simulink model "induction_motor_drive"  (Simulink 5.0)
settings: Solver=ode23tb  SolverMode=SingleTasking  StartTime=0.0  StopTime=2  MaxStep=10e-6  RelTol=1e-4
undefined symbols (not defined in the file): sigbuilder_block
libraries: powerlib2 x6
settings Model: Creator=Oros  ExtModeTrigMode=oneshot  ExtModeArmWhenConnect=off  ExternalInput=[]  TimeSaveName=t  SaveOutput=off  LimitDataPoints=off  UnconnectedInputMsg=none  UnconnectedOutputMsg=none  BlockReductionOpt=off  BooleanDataType=off  RTWTemplateMakefile=grt_unix.tmf

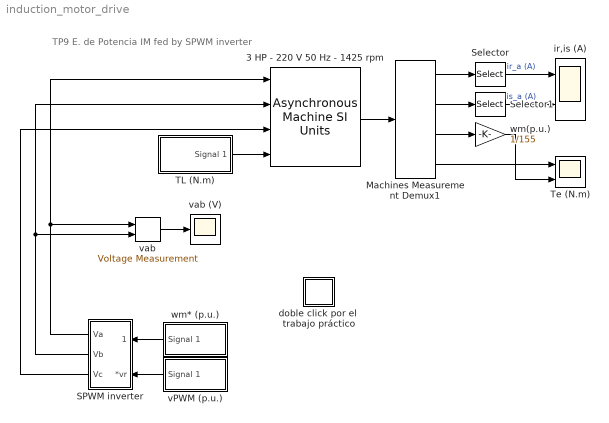
== system induction_motor_drive ==
  note: TP9 E. de Potencia
      | IM fed by SPWM inverter
  3 HP - 220 V 50 Hz - 1425 rpm : powerlib2/Machines/Asynchronous Machine SI Units  Tag=PoWeRsYsTeMbLoCk  rotType=Squirrel-cage  ctrl=Stationary  x1=[ 5*746, 220, 50 ]  x2="[ 0.435  2*2.0e-3 ]"  x3="[ 0.816  2.0e-3 ]"  x4=69.31e-3  x5="[ 0.089  0  2 ]"  x6="[ 1,0   0,0,0   0,0,0 ]"  PSBOutputType=1110  iounits=1  LoadFlowParameters=0
  Machines Measurement Demux1 : powerlib2/Machines/Machines Measurement Demux  machType=Asynchronous  ssm1=on  ssm2=on  ssm3=on  ssm4=on  ssm5=on  ssm6=on  sm1=off  sm2=on  sm3=off  sm4=off  sm5=off  sm6=on  sm7=off  sm8=on  sm9=off  sm10=off  sm11=off  sm115=off  sm12=off  sm13=off  sm14=off  asm1=on  asm2=off  asm3=off  asm4=off  asm5=on  asm6=off  asm7=off  asm8=off  asm9=on  asm10=on  asm11=off  pmsm1=on  pmsm2=on  pmsm3=on  pmsm4=on  pmsm5=on  pmsm6=on  lastType=1
  SPWM inverter : Subsystem  Orientation=left
  Selector : Selector  InputPortWidth=3
  Selector1 : Selector  InputPortWidth=3
  TL (N.m) : Subsystem  Tag=STV Subsys  StartFcn=sigbuilder_block('start');  StopFcn=sigbuilder_block('stop');  ClipboardFcn=sigbuilder_block('clipboard');  mask(Sigbuilder block){}
      mask help: Sigbuilder GUI
      mask init:
      | if ~strcmp(get_param(bdroot(gcb),'SimulationStatus'),'stopped') tuvar = sigbuilder_block('maskInit'); end
      settings: CopyFcn=sigbuilder_block('copy');  DeleteFcn=sigbuilder_block('delete');  ModelCloseFcn=sigbuilder_block('modelClose');  PreSaveFcn=sigbuilder_block('preSave');  NameChangeFcn=sigbuilder_block('namechange');  OpenFcn=sigbuilder_block('open',[78 40.5 391.5 291 ]);  CloseFcn=sigbuilder_block('close');
      mask Display: plot(0,0,100,100,[10,10,40,40,10],[80,20,20,80,80],[40,10],[50,50], [40,27,10],[65,72,56],[40,25,25,10],[28,28,43,43]);
  Te (N.m) : Scope  NumInputPorts=2
      settings: YMin=-125~0.05  YMax=200~1.05  DataFormat=Structure
  doble click por el  trabajo práctico : Subsystem
      mask Display: disp('?')
  ir,is (A) : Scope  NumInputPorts=2
      settings: YMin=-100~-80  YMax=110~100  DataFormat=Structure
  vPWM (p.u.) : Subsystem  Tag=STV Subsys  Orientation=left  StartFcn=sigbuilder_block('start');  StopFcn=sigbuilder_block('stop');  ClipboardFcn=sigbuilder_block('clipboard');  mask(Sigbuilder block){}
      mask help: Sigbuilder GUI
      mask init:
      | if ~strcmp(get_param(bdroot(gcb),'SimulationStatus'),'stopped') tuvar = sigbuilder_block('maskInit'); end
      settings: CopyFcn=sigbuilder_block('copy');  DeleteFcn=sigbuilder_block('delete');  ModelCloseFcn=sigbuilder_block('modelClose');  PreSaveFcn=sigbuilder_block('preSave');  NameChangeFcn=sigbuilder_block('namechange');  OpenFcn=sigbuilder_block('open',[78 40.5 391.5 291 ]);  CloseFcn=sigbuilder_block('close');
      mask Display: plot(0,0,100,100,[10,10,40,40,10],[80,20,20,80,80],[40,10],[50,50], [40,27,10],[65,72,56],[40,25,25,10],[28,28,43,43]);
  vab : powerlib2/Measurements/Voltage Measurement  Tag=PoWeRsYsTeMmEaSuReMeNt  PhasorSimulation=off  OutputType=Magnitude  PSBOutputType=0  PSBequivalent=1
  vab (V) : Scope
      settings: YMin=-400  YMax=400  DataFormat=Structure
  wm(p.u.) : Gain  Gain=1/155  SaturateOnIntegerOverflow=on
  wm* (p.u.) : Subsystem  Tag=STV Subsys  Orientation=left  StartFcn=sigbuilder_block('start');  StopFcn=sigbuilder_block('stop');  ClipboardFcn=sigbuilder_block('clipboard');  mask(Sigbuilder block){}
      mask help: Sigbuilder GUI
      mask init:
      | if ~strcmp(get_param(bdroot(gcb),'SimulationStatus'),'stopped') tuvar = sigbuilder_block('maskInit'); end
      settings: CopyFcn=sigbuilder_block('copy');  DeleteFcn=sigbuilder_block('delete');  ModelCloseFcn=sigbuilder_block('modelClose');  PreSaveFcn=sigbuilder_block('preSave');  NameChangeFcn=sigbuilder_block('namechange');  OpenFcn=sigbuilder_block('open',[78 40.5 391.5 291 ]);  CloseFcn=sigbuilder_block('close');
      mask Display: plot(0,0,100,100,[10,10,40,40,10],[80,20,20,80,80],[40,10],[50,50], [40,27,10],[65,72,56],[40,25,25,10],[28,28,43,43]);
  wires:
  SPWM inverter/1(Va) -> vab/1, 3 HP - 220 V 50 Hz - 1425 rpm/1
  SPWM inverter/2(Vb) -> vab/2, 3 HP - 220 V 50 Hz - 1425 rpm/2
  vab/1 -> vab (V)/1
  Machines Measurement Demux1/1 -> Selector/1
  Machines Measurement Demux1/3 -> wm(p.u.)/1
  Machines Measurement Demux1/4 -> Te (N.m)/1
  Machines Measurement Demux1/2 -> Selector1/1
  Selector/1 -> ir,is (A)/1  "ir_a (A)"
  Selector1/1 -> ir,is (A)/2  "is_a (A)"
  3 HP - 220 V 50 Hz - 1425 rpm/1 -> Machines Measurement Demux1/1
  SPWM inverter/3(Vc) -> 3 HP - 220 V 50 Hz - 1425 rpm/3
  wm* (p.u.)/1(Signal 1) -> SPWM inverter/1(*wr)
  vPWM (p.u.)/1(Signal 1) -> SPWM inverter/2(*vr)
  wm(p.u.)/1 -> Te (N.m)/2
  TL (N.m)/1(Signal 1) -> 3 HP - 220 V 50 Hz - 1425 rpm/4

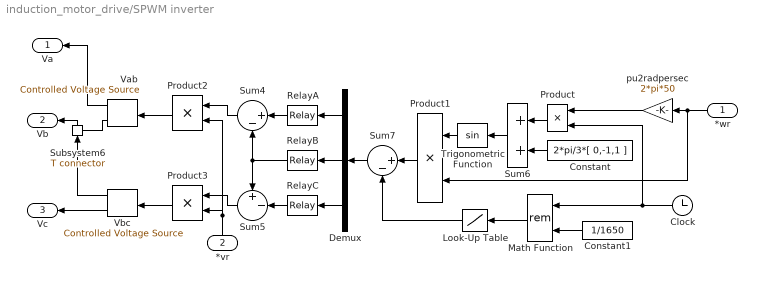
== system induction_motor_drive/SPWM inverter ==
  *wr : Inport  Orientation=left
  *vr : Inport  Orientation=up  Port=2
  Clock : Clock
      settings: Decimation=10
  Constant : Constant  Orientation=left  Value=2*pi/3*[ 0,-1,1 ]
  Constant1 : Constant  Orientation=left  Value=1/1650
  Demux : Demux  Orientation=left  Outputs=3
  Look-Up Table : Lookup  Orientation=left  InputValues="[0 0.25  0.75  1] / 1650"  OutputValues="[0  1  -1  0]"  SaturateOnIntegerOverflow=on
  Math Function : Math  Orientation=left  Operator=rem
  Product : Product  Orientation=left  SaturateOnIntegerOverflow=on  InputSameDT=on
  Product1 : Product  Orientation=left  SaturateOnIntegerOverflow=on  InputSameDT=on
  Product2 : Product  Orientation=left  SaturateOnIntegerOverflow=on
  Product3 : Product  Orientation=left  SaturateOnIntegerOverflow=on
  RelayA : Relay  Orientation=left  OnSwitchValue=0  OffSwitchValue=0  OnOutputValue=220*sqrt(2/3)  OffOutputValue=-220*sqrt(2/3)
  RelayB : Relay  Orientation=left  OnSwitchValue=0  OffSwitchValue=0  OnOutputValue=220*sqrt(2/3)  OffOutputValue=-220*sqrt(2/3)
  RelayC : Relay  Orientation=left  OnSwitchValue=0  OffSwitchValue=0  OnOutputValue=220*sqrt(2/3)  OffOutputValue=-220*sqrt(2/3)
  Subsystem6 : powerlib2/Connectors/T connector  Tag=PoWeRsYsTeMbLoCk  Orientation=up  PSBOutputType=1
  Sum4 : Sum  Orientation=left  Inputs=|+-  SaturateOnIntegerOverflow=on  InputSameDT=on
  Sum5 : Sum  Orientation=left  Inputs=+-|  SaturateOnIntegerOverflow=on  InputSameDT=on
  Sum6 : Sum  Orientation=left  SaturateOnIntegerOverflow=on  InputSameDT=on
  Sum7 : Sum  Orientation=left  Inputs=|+-  SaturateOnIntegerOverflow=on  InputSameDT=on
  Trigonometric Function : Trigonometry  Orientation=left
  Vab : powerlib2/Electrical Sources/Controlled Voltage Source  Tag=PoWeRsYsTeMbLoCk  Orientation=left  initsrc=on  srctyp=AC  iv=0  iph=0  ifreq=0  mesure=None  PSBOutputType=11
  Vbc : powerlib2/Electrical Sources/Controlled Voltage Source  Tag=PoWeRsYsTeMbLoCk  Orientation=left  initsrc=on  srctyp=AC  iv=0  iph=0  ifreq=0  mesure=None  PSBOutputType=11
  pu2radpersec : Gain  Orientation=left  Gain=2*pi*50  SaturateOnIntegerOverflow=on
  Va : Outport  Orientation=left
  Vb : Outport  Orientation=left  Port=2
  Vc : Outport  Orientation=left  Port=3
  wires:
  RelayA/1 -> Sum4/1
  RelayC/1 -> Sum5/2
  RelayB/1 -> Sum5/1, Sum4/2
  Demux/2 -> RelayB/1
  Demux/3 -> RelayC/1
  Demux/1 -> RelayA/1
  Sum7/1 -> Demux/1
  pu2radpersec/1 -> Product/1
  Sum6/1 -> Trigonometric Function/1
  Trigonometric Function/1 -> Product1/1
  Product1/1 -> Sum7/1
  *wr/1 -> Product1/2, pu2radpersec/1
  Look-Up Table/1 -> Sum7/2
  Clock/1 -> Product/2, Math Function/1
  Math Function/1 -> Look-Up Table/1
  Constant1/1 -> Math Function/2
  Product/1 -> Sum6/1
  Constant/1 -> Sum6/2
  Product2/1 -> Vab/1
  Sum4/1 -> Product2/1
  Product3/1 -> Vbc/1
  Sum5/1 -> Product3/1
  *vr/1 -> Product3/2, Product2/2
  Vab/1 -> Va/1
  Vbc/2 -> Vc/1
  Vab/2 -> Subsystem6/Enable
  Vbc/1 -> Subsystem6/1
  Subsystem6/1 -> Vb/1

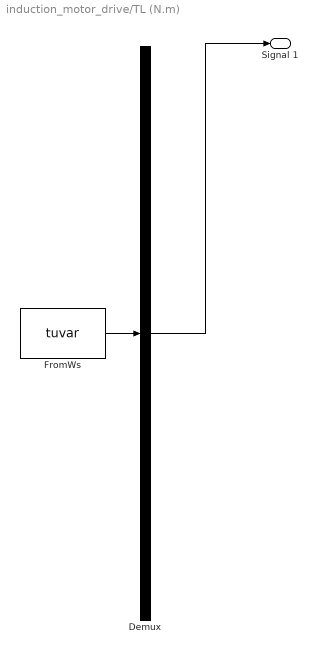
== system induction_motor_drive/TL (N.m) ==
  Demux : Demux  Tag=STV Demux  Outputs=1
  FromWs : FromWorkspace  Tag=STV FromWs  VariableName=tuvar  SampleTime=0  SigBuilderData=DataTag0
      SigBuilderData=|
      | channels.label = 'Signal 1'
      | channels.allXData = {[0 0.1 0.1 1 1 2]}
      | channels.allYData = {[5.9 5.9 5.95 5.95 20 20]}
      | dataSet.timeRange = [0 2]
      | dataSet.name = 'Group 1'
  Signal 1 : Outport  Tag=STV Outport
  wires:
  Demux/1 -> Signal 1/1
  FromWs/1 -> Demux/1

== system induction_motor_drive/doble click por el  trabajo práctico ==
  note: TP 9; Case study II: Induction motor v/f drive
  note: Measurements
  note: Conclusion
  note: Womework
  note: Circuit dscription
  note: El motor de AC está alimentado por un convertidor de AC, donde se puede variar la relación v/f
      | La carga mecánica está caracterizada por un escalón de carga TL.
  note: Ejecute la simulación (Matlab 6.5 o superior). Observe en el osciloscopio la velocidad y el par temporales.
      | Observe en el osciloscopio las corrientes ir, is y la tensión Vab
  note: Realizar el siguiente análisis:
      |
      | a) interpretar el circuito, la señal de entrada y la variación de par de carga
      | b) correr el circuito de Simulink
      | c) imprimir los resultados
      | d) interpretar los resultados, en base a la variación de la señal de
      | referencia y variación del par de carga TL
      | e) analizar la variación de Vab
  note: Escriba las conclusiones
      |
      | a) acerca del modo de arranque
      | b) acerca de la ecuación general de par Te=TL+J*d(wm)/dt
      | c) acerca de la relación velocidad/
      | c) generales (otros)

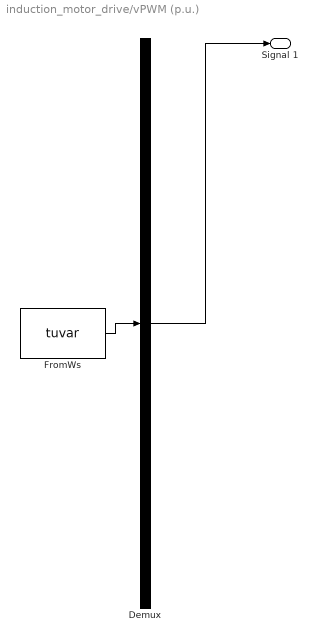
== system induction_motor_drive/vPWM (p.u.) ==
  Demux : Demux  Tag=STV Demux  Outputs=1
  FromWs : FromWorkspace  Tag=STV FromWs  VariableName=tuvar  SampleTime=0  SigBuilderData=DataTag1
      SigBuilderData=|
      | channels.label = 'Signal 1'
      | channels.allXData = {[0 0.1 0.1 0.505 0.505 1 2]}
      | channels.allYData = {[0.51 0.51 1 1 0.705 0.705 0.705]}
      | dataSet.timeRange = [0 2]
      | dataSet.name = 'Group 1'
  Signal 1 : Outport  Tag=STV Outport
  wires:
  FromWs/1 -> Demux/1
  Demux/1 -> Signal 1/1

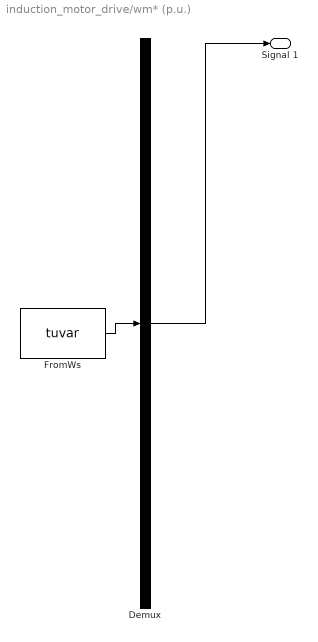
== system induction_motor_drive/wm* (p.u.) ==
  Demux : Demux  Tag=STV Demux  Outputs=1
  FromWs : FromWorkspace  Tag=STV FromWs  VariableName=tuvar  SampleTime=0  SigBuilderData=DataTag2
      SigBuilderData=|
      | channels.label = 'Signal 1'
      | channels.allXData = {[0 0.1 0.1 0.505 0.505 2]}
      | channels.allYData = {[0.51 0.51 0.995 0.995 0.705 0.705]}
      | dataSet.timeRange = [0 2]
      | dataSet.name = 'Group 1'
  Signal 1 : Outport  Tag=STV Outport
  wires:
  Demux/1 -> Signal 1/1
  FromWs/1 -> Demux/1
